simulink model "swinguplisan1122"  (R2021a)
settings: Solver=ode3  StartTime=0.0  StopTime=30  FixedStep=0.005  RelTol=1e-3
undefined symbols (not defined in the file or in its folder): DiscIntNeverNeededParam
libraries: simulink x1
settings Model: EnablePacing=on  PacingRate=0.630000  Creator=zju308  LastModifiedBy=zju308
settings SolverCC: ZeroCrossAlgorithm=Adaptive
settings DebuggingCC: IgnoredZcDiagnostic=none

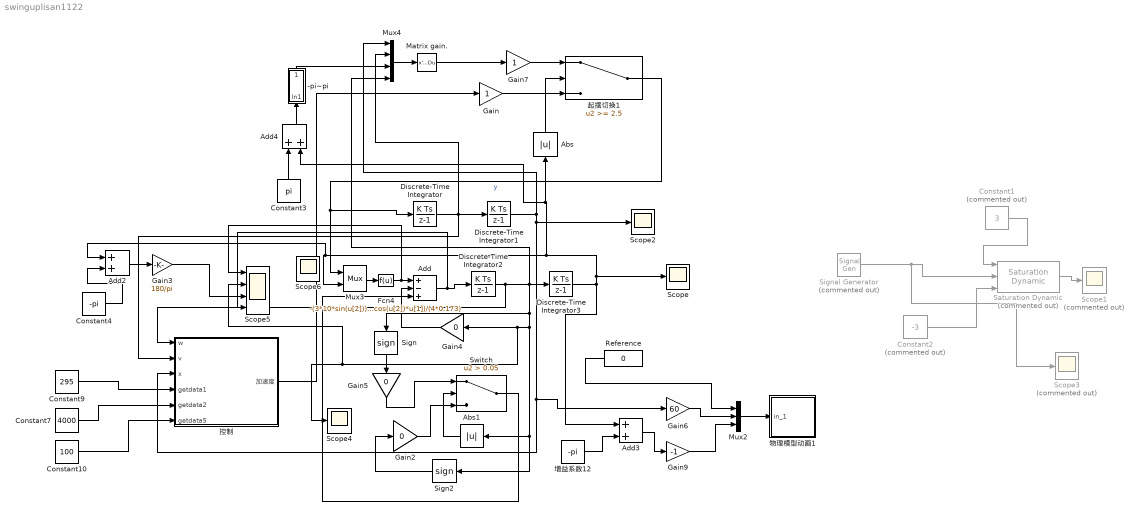
== system swinguplisan1122 ==
  " -pi~pi" : Subsystem  mask(Change){}
      mask help:
      | Change input signal between -pi and pi in 2*pi period.
      | Block input:
      |     any double.
      | Block output:
      |     between -pi and pi.
      | eg:
      |     If input is 1.5*pi, then output is -0.5*pi.
      mask Display: plot([0:0.01:2*pi],sin([0:0.01:2*pi]));
  Abs : Abs
  Abs1 : Abs
  Add : Sum  Inputs=+-+
  Add2 : Sum
  Add3 : Sum
  Add4 : Sum
  Constant1 : Constant  Commented=on  Value=3
  Constant10 : Constant  Value=100
  Constant2 : Constant  Commented=on  Value=-3
  Constant3 : Constant  Value=pi
  Constant4 : Constant  Value=-pi
  Constant7 : Constant  Value=4000
  Constant9 : Constant  Value=295
  Discrete-Time Integrator{,1..3} (4 alike) : DiscreteIntegrator  SampleTime=-1  ICPrevOutput=DiscIntNeverNeededParam  ICPrevScaledInput=DiscIntNeverNeededParam
  Fcn4 : Fcn  Expr=-(3*10*sin(u[2]))/(4*0.173)-(3*cos(u[2])*u[1])/(4*0.173)
  Gain : Gain
  Gain2 : Gain  Gain=0
  Gain3 : Gain  Gain=180/pi
  Gain4 : Gain  Gain=0
  Gain5 : Gain  Gain=0
  Gain6 : Gain  Gain=60
  Gain7 : Gain
  Gain9 : Gain  Gain=-1
  Matrix gain. : StateSpace  A=[]  B=[]  C=[]  D=K  InitialCondition=0  mask(Matrix gain){K=[18 14 -57 -8]}
      mask prompts: K "Gain matrix:"
      mask help: Matrix Gain:
      mask Help: Multiplies input vector by entered matrix to produce output vector.
      mask Display: disp('LQR')
  Mux2 : Mux  Inputs=3
  Mux3 : Mux  Inputs=2
  Mux4 : Mux
  Reference : Constant  Value=0
  Saturation Dynamic : simulink/Discontinuities/Saturation Dynamic  Commented=on  OutMin=[]  OutMax=[]  OutDataTypeStr=Inherit: Same as second input  OutDataType=fixdt(1, 16)  OutScaling=2^-10  DoSatur=off
  Scope{,2,4,6} (4 alike) : Scope
  Scope1 : Scope  Commented=on
  Scope3 : Scope  Commented=on
  Scope5 : Scope  NumInputPorts=4
  Sign : Signum
  Sign2 : Signum
  Signal Generator : SignalGenerator  Commented=on  Amplitude=10  Units=rad/sec
  Switch : Switch  Criteria=u2 > Threshold  Threshold=0.05
  增益系数12 : Constant  Value=-pi
  控制 : Subsystem
  物理模型动画1 : Subsystem  mask(Pendulum plot){RefBlock=Reference}
      mask prompts: RefBlock "DC reference signal block name:"
      mask help: Pendulum plot
      mask Help: Pendulum animation function using Handle graphics.
      mask Display: plot([-10 10],[0 0],[-2 -2 2 2],[0 1 1 0],[0 3],[1 5])
  起摆切换1 : Switch  Threshold=2.5
  wires:
  Gain6/1 -> Mux2/2
  Add3/1 -> Gain9/1
  Mux2/1 -> 物理模型动画1/1(in_1)
  增益系数12/1 -> Add3/2
  Reference/1 -> Mux2/1
  Mux3/1 -> Fcn4/1
  Gain9/1 -> Mux2/3
  Constant7/1 -> 控制/5(getdata2)
  Constant9/1 -> 控制/4(getdata1)
  Constant10/1 -> 控制/6(getdata5)
  Mux4/1 -> Matrix gain./1
  Discrete-Time Integrator/1 -> Discrete-Time Integrator1/1, Mux4/2, 控制/2(v)
  控制/1(加速度) -> Gain/1
  Abs/1 -> 起摆切换1/2
  " -pi~pi"/1(Out1) -> Mux4/3
  Add4/1 -> " -pi~pi"/1(In1)
  Constant3/1 -> Add4/1
  Discrete-Time Integrator1/1 -> Scope2/1, 控制/3(x), Gain6/1, Mux4/1
  Fcn4/1 -> Scope5/1, Add/1
  Add/1 -> Scope5/4, Discrete-Time Integrator2/1
  Discrete-Time Integrator3/1 -> Add2/1, Mux3/2, Add4/2, Abs/1, Scope/1, Add3/1
  起摆切换1/1 -> Discrete-Time Integrator/1, Mux3/1  "y"
  Switch/1 -> Add/3
  Gain4/1 -> Add/2
  Gain/1 -> 起摆切换1/3
  Gain7/1 -> 起摆切换1/1
  Signal Generator/1 -> Scope3/1, Saturation Dynamic/2
  Constant1/1 -> Saturation Dynamic/1
  Constant2/1 -> Saturation Dynamic/3
  Saturation Dynamic/1 -> Scope1/1
  Abs1/1 -> Switch/2
  Discrete-Time Integrator2/1 -> 控制/1(w), Discrete-Time Integrator3/1, Sign2/1, Abs1/1, Scope5/2, Scope4/1, Gain4/1, Sign/1, Mux4/4
  Sign/1 -> Gain5/1
  Gain5/1 -> Switch/1
  Gain2/1 -> Switch/3
  Add2/1 -> Gain3/1
  Constant4/1 -> Add2/2
  Gain3/1 -> Scope5/3
  Sign2/1 -> Gain2/1
  Matrix gain./1 -> Gain7/1

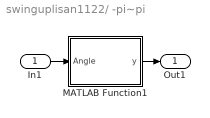
== system swinguplisan1122/ -pi~pi ==
  In1 : Inport
  MATLAB Function1 : MATLAB Function  TreatAsAtomicUnit=on
  Out1 : Outport  VectorParamsAs1DForOutWhenUnconnected=off
  wires:
  MATLAB Function1/1(y) -> Out1/1
  In1/1 -> MATLAB Function1/1(Angle)

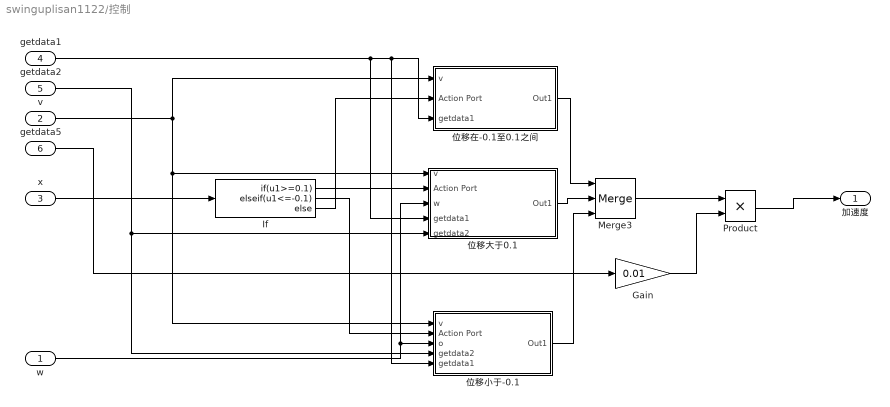
== system swinguplisan1122/控制 ==
  w : Inport
  v : Inport  Port=2
  x : Inport  Port=3
  getdata1 : Inport  Port=4
  getdata2 : Inport  Port=5
  getdata5 : Inport  Port=6
  Gain : Gain  Gain=0.01
  If : If  IfExpression=u1>=0.1  ElseIfExpressions=u1<=-0.1
  Merge3 : Merge  Inputs=3
  Product : Product
  位移在-0.1至0.1之间 : Subsystem
  位移大于0.1 : Subsystem
  位移小于-0.1 : Subsystem
  加速度 : Outport
  wires:
  w/1 -> 位移大于0.1/3(w), 位移小于-0.1/3(o)
  v/1 -> 位移小于-0.1/1(v), 位移大于0.1/1(v), 位移在-0.1至0.1之间/1(v)
  位移大于0.1/1(Out1) -> Merge3/2
  位移在-0.1至0.1之间/1(Out1) -> Merge3/1
  位移小于-0.1/1(Out1) -> Merge3/3
  If/1 -> 位移大于0.1/2(Action Port)
  x/1 -> If/1
  If/3 -> 位移在-0.1至0.1之间/2(Action Port)
  If/2 -> 位移小于-0.1/2(Action Port)
  getdata1/1 -> 位移在-0.1至0.1之间/3(getdata1), 位移小于-0.1/5(getdata1), 位移大于0.1/4(getdata1)
  getdata2/1 -> 位移小于-0.1/4(getdata2), 位移大于0.1/5(getdata2)
  Gain/1 -> Product/2
  getdata5/1 -> Gain/1
  Merge3/1 -> Product/1
  Product/1 -> 加速度/1

== system swinguplisan1122/物理模型动画1 ==
  in_1 : Inport
  S-function : S-Function  FunctionName=UpPendAnim  Parameters=RefBlock  SFunctionDeploymentMode=off  EnableBusSupport=off
      settings: DeleteFcn=pendan([],[],[],'DeleteBlock');
  wires:
  in_1/1 -> S-function/1

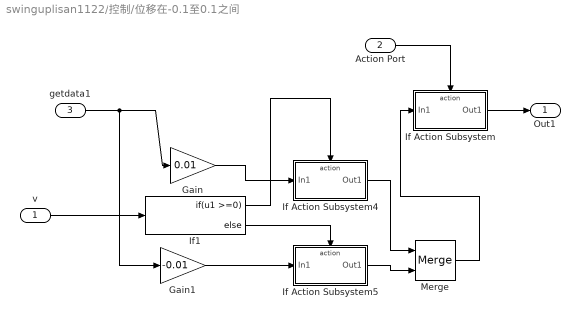
== system swinguplisan1122/控制/位移在-0.1至0.1之间 ==
  v : Inport
  Action Port : Inport  Port=2
  getdata1 : Inport  Port=3
  Gain : Gain  Gain=0.01
  Gain1 : Gain  Gain=-0.01
  If Action Subsystem : Subsystem  TreatAsAtomicUnit=on
  If Action Subsystem4 : Subsystem  TreatAsAtomicUnit=on
  If Action Subsystem5 : Subsystem  TreatAsAtomicUnit=on
  If1 : If  IfExpression=u1 >=0
  Merge : Merge
  Out1 : Outport
  wires:
  If Action Subsystem4/1(Out1) -> Merge/1
  Gain1/1 -> If Action Subsystem5/1(In1)
  If1/2 -> If Action Subsystem5/Action
  If Action Subsystem5/1(Out1) -> Merge/2
  Gain/1 -> If Action Subsystem4/1(In1)
  If1/1 -> If Action Subsystem4/Action
  Action Port/1 -> If Action Subsystem/Action
  Merge/1 -> If Action Subsystem/1(In1)
  v/1 -> If1/1
  If Action Subsystem/1(Out1) -> Out1/1
  getdata1/1 -> Gain1/1, Gain/1

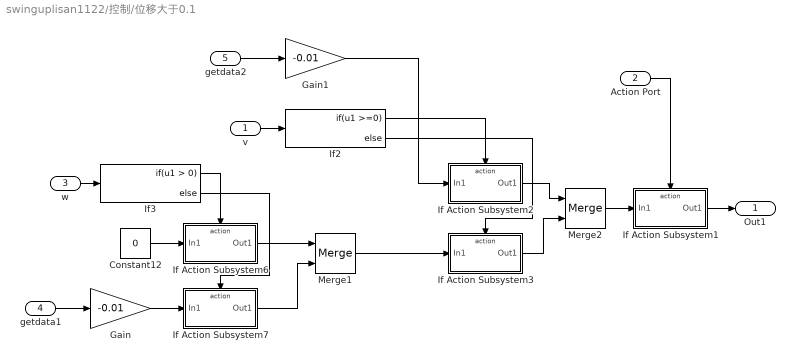
== system swinguplisan1122/控制/位移大于0.1 ==
  v : Inport
  Action Port : Inport  Port=2
  w : Inport  Port=3
  getdata1 : Inport  Port=4
  getdata2 : Inport  Port=5
  Constant12 : Constant  Value=0
  Gain : Gain  Gain=-0.01
  Gain1 : Gain  Gain=-0.01
  If Action Subsystem1 : Subsystem  TreatAsAtomicUnit=on
  If Action Subsystem2 : Subsystem  TreatAsAtomicUnit=on
  If Action Subsystem3 : Subsystem  TreatAsAtomicUnit=on
  If Action Subsystem6 : Subsystem  TreatAsAtomicUnit=on
  If Action Subsystem7 : Subsystem  TreatAsAtomicUnit=on
  If2 : If  IfExpression=u1 >=0
  If3 : If
  Merge1 : Merge
  Merge2 : Merge
  Out1 : Outport
  wires:
  If Action Subsystem1/1(Out1) -> Out1/1
  Gain1/1 -> If Action Subsystem2/1(In1)
  Merge2/1 -> If Action Subsystem1/1(In1)
  If Action Subsystem6/1(Out1) -> Merge1/1
  If2/1 -> If Action Subsystem2/Action
  If Action Subsystem3/1(Out1) -> Merge2/2
  If3/1 -> If Action Subsystem6/Action
  Action Port/1 -> If Action Subsystem1/Action
  Constant12/1 -> If Action Subsystem6/1(In1)
  Merge1/1 -> If Action Subsystem3/1(In1)
  If Action Subsystem7/1(Out1) -> Merge1/2
  If Action Subsystem2/1(Out1) -> Merge2/1
  Gain/1 -> If Action Subsystem7/1(In1)
  If2/2 -> If Action Subsystem3/Action
  If3/2 -> If Action Subsystem7/Action
  v/1 -> If2/1
  w/1 -> If3/1
  getdata1/1 -> Gain/1
  getdata2/1 -> Gain1/1

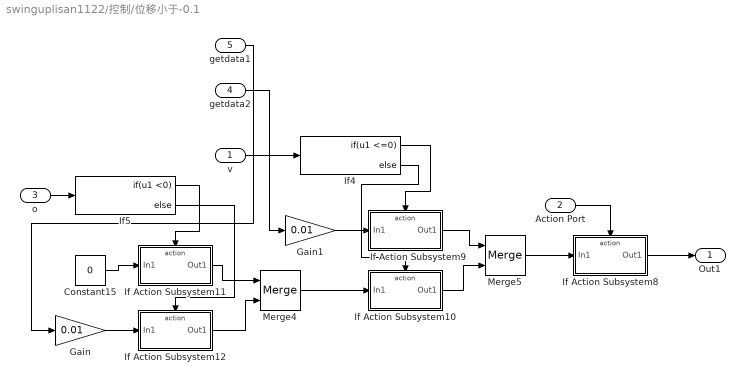
== system swinguplisan1122/控制/位移小于-0.1 ==
  v : Inport
  Action Port : Inport  Port=2
  o : Inport  Port=3
  getdata2 : Inport  Port=4
  getdata1 : Inport  Port=5
  Constant15 : Constant  Value=0
  Gain : Gain  Gain=0.01
  Gain1 : Gain  Gain=0.01
  If Action Subsystem10 : Subsystem  TreatAsAtomicUnit=on
  If Action Subsystem11 : Subsystem  TreatAsAtomicUnit=on
  If Action Subsystem12 : Subsystem  TreatAsAtomicUnit=on
  If Action Subsystem8 : Subsystem  TreatAsAtomicUnit=on
  If Action Subsystem9 : Subsystem  TreatAsAtomicUnit=on
  If4 : If  IfExpression=u1 <=0
  If5 : If  IfExpression=u1 <0
  Merge4 : Merge
  Merge5 : Merge
  Out1 : Outport
  wires:
  Gain/1 -> If Action Subsystem12/1(In1)
  Merge5/1 -> If Action Subsystem8/1(In1)
  Constant15/1 -> If Action Subsystem11/1(In1)
  If Action Subsystem9/1(Out1) -> Merge5/1
  If4/2 -> If Action Subsystem10/Action
  If5/1 -> If Action Subsystem11/Action
  If5/2 -> If Action Subsystem12/Action
  If Action Subsystem8/1(Out1) -> Out1/1
  If Action Subsystem12/1(Out1) -> Merge4/2
  If Action Subsystem11/1(Out1) -> Merge4/1
  Merge4/1 -> If Action Subsystem10/1(In1)
  If4/1 -> If Action Subsystem9/Action
  v/1 -> If4/1
  If Action Subsystem10/1(Out1) -> Merge5/2
  Gain1/1 -> If Action Subsystem9/1(In1)
  Action Port/1 -> If Action Subsystem8/Action
  o/1 -> If5/1
  getdata1/1 -> Gain/1
  getdata2/1 -> Gain1/1

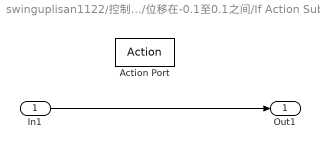
== system swinguplisan1122/控制/位移在-0.1至0.1之间/If Action Subsystem ==
  In1 : Inport
  Action Port : ActionPort  ActionPortLabel=else
  Out1 : Outport
  wires:
  In1/1 -> Out1/1

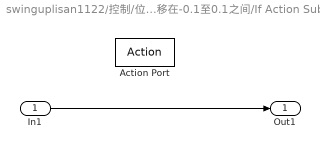
== system swinguplisan1122/控制/位移在-0.1至0.1之间/If Action Subsystem4 ==
  In1 : Inport
  Action Port : ActionPort  ActionPortLabel=if(u1 >=0)
  Out1 : Outport
  wires:
  In1/1 -> Out1/1

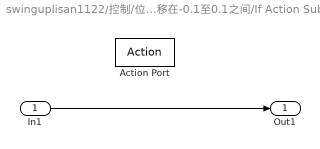
== system swinguplisan1122/控制/位移在-0.1至0.1之间/If Action Subsystem5 ==
  In1 : Inport
  Action Port : ActionPort  ActionPortLabel=else
  Out1 : Outport
  wires:
  In1/1 -> Out1/1

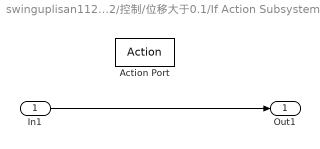
== system swinguplisan1122/控制/位移大于0.1/If Action Subsystem1 ==
  In1 : Inport
  Action Port : ActionPort  ActionPortLabel=if(u1>=0.1)
  Out1 : Outport
  wires:
  In1/1 -> Out1/1

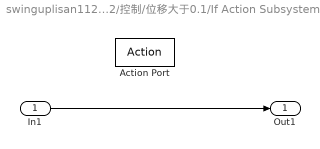
== system swinguplisan1122/控制/位移大于0.1/If Action Subsystem2 ==
  In1 : Inport
  Action Port : ActionPort  ActionPortLabel=if(u1 >=0)
  Out1 : Outport
  wires:
  In1/1 -> Out1/1

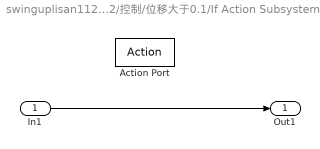
== system swinguplisan1122/控制/位移大于0.1/If Action Subsystem3 ==
  In1 : Inport
  Action Port : ActionPort  ActionPortLabel=else
  Out1 : Outport
  wires:
  In1/1 -> Out1/1

== system swinguplisan1122/控制/位移大于0.1/If Action Subsystem6 ==
  In1 : Inport
  Action Port : ActionPort  ActionPortLabel=if(u1 > 0)
  Out1 : Outport
  wires:
  In1/1 -> Out1/1

== system swinguplisan1122/控制/位移大于0.1/If Action Subsystem7 ==
  In1 : Inport
  Action Port : ActionPort  ActionPortLabel=else
  Out1 : Outport
  wires:
  In1/1 -> Out1/1

== system swinguplisan1122/控制/位移小于-0.1/If Action Subsystem10 ==
  In1 : Inport
  Action Port : ActionPort  ActionPortLabel=else
  Out1 : Outport
  wires:
  In1/1 -> Out1/1

== system swinguplisan1122/控制/位移小于-0.1/If Action Subsystem11 ==
  In1 : Inport
  Action Port : ActionPort  ActionPortLabel=if(u1 <0)
  Out1 : Outport
  wires:
  In1/1 -> Out1/1

== system swinguplisan1122/控制/位移小于-0.1/If Action Subsystem12 ==
  In1 : Inport
  Action Port : ActionPort  ActionPortLabel=else
  Out1 : Outport
  wires:
  In1/1 -> Out1/1

== system swinguplisan1122/控制/位移小于-0.1/If Action Subsystem8 ==
  In1 : Inport
  Action Port : ActionPort  ActionPortLabel=elseif(u1<=-0.1)
  Out1 : Outport
  wires:
  In1/1 -> Out1/1

== system swinguplisan1122/控制/位移小于-0.1/If Action Subsystem9 ==
  In1 : Inport
  Action Port : ActionPort  ActionPortLabel=if(u1 <=0)
  Out1 : Outport
  wires:
  In1/1 -> Out1/1

== matlab function swinguplisan1122/ -pi~pi/MATLAB Function1 ==
  data: Angle input; y output
function y = Change(Angle)
%#codegen
    y=0;
    while ( Angle > pi) 
        Angle = Angle-2 * pi;
    end
    while (Angle <= -pi) 
        Angle = Angle+2 * pi;
    end 
    y=Angle+y;
end
